simulink model "untitled"  (R2024b)
settings: Solver=VariableStepAuto  StartTime=0.0  StopTime=10.0  RelTol=1e-3
settings Model: Creator=yugan  LastModifiedBy=yugan
settings DebuggingCC: AlgebraicLoopMsg=none

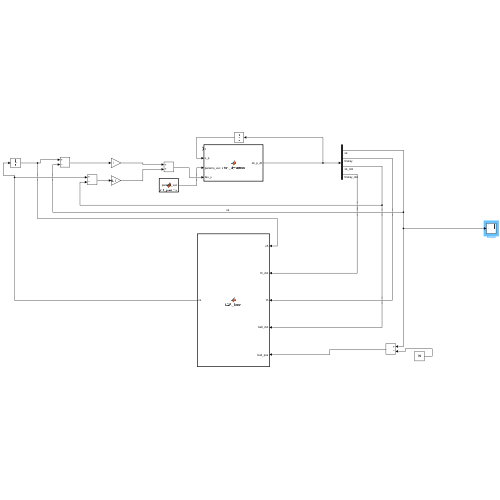
[thumbnail: Simulink's stored preview of the top-level diagram]
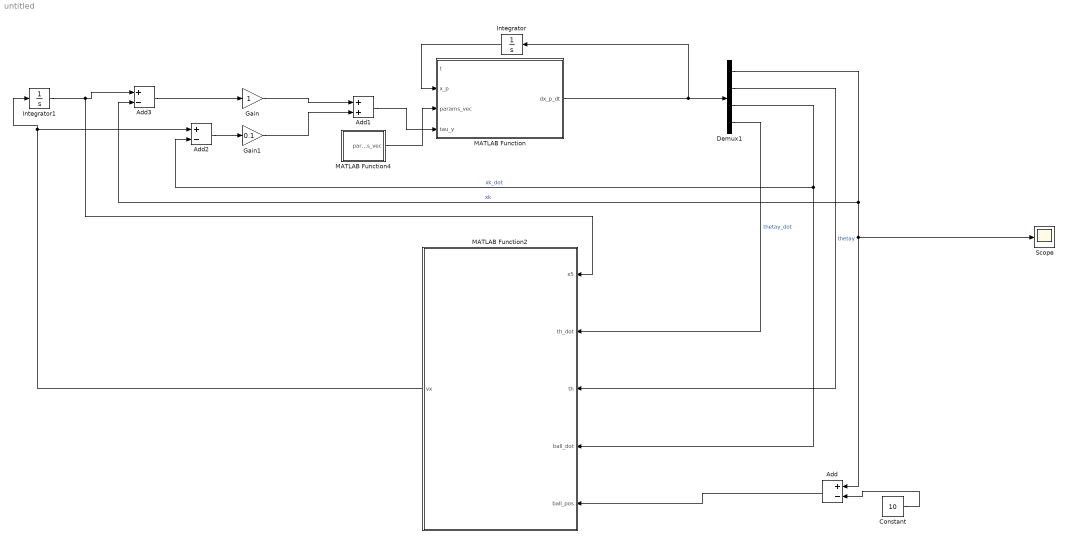
== system untitled ==
  Add : Sum  Inputs=+-
  Add1 : Sum
  Add2 : Sum  Inputs=+-
  Add3 : Sum  Inputs=+-
  Constant : Constant  Value=10
  Demux1 : Demux
  Gain : Gain
  Gain1 : Gain  Gain=0.1
  Integrator : Integrator  InitialCondition=[0; 0; 0; 0]
  Integrator1 : Integrator
  MATLAB Function : MATLAB Function  TreatAsAtomicUnit=on
  MATLAB Function2 : MATLAB Function  TreatAsAtomicUnit=on
  MATLAB Function4 : MATLAB Function  TreatAsAtomicUnit=on
  Scope : Scope
  wires:
  Integrator/1 -> MATLAB Function/2(x_p)
  MATLAB Function/1(dx_p_dt) -> Demux1/1, Integrator/1
  Demux1/1 -> Add3/2, Scope/1, Add/1  "xk"
  Add/1 -> MATLAB Function2/5(ball_pos)
  Constant/1 -> Add/2
  Demux1/2 -> MATLAB Function2/3(th)  "thetay"
  Demux1/3 -> MATLAB Function2/4(ball_dot), Add2/2  "xk_dot"
  Demux1/4 -> MATLAB Function2/2(th_dot)  "thetay_dot"
  Add1/1 -> MATLAB Function/4(tau_y)
  MATLAB Function4/1(params_vec) -> MATLAB Function/3(params_vec)
  Gain/1 -> Add1/1
  Gain1/1 -> Add1/2
  Add2/1 -> Gain1/1
  Add3/1 -> Gain/1
  MATLAB Function2/1(vx) -> Add2/1, Integrator1/1
  Integrator1/1 -> MATLAB Function2/1(x5), Add3/1

== matlab function untitled/MATLAB Function ==
  data: t input; dx_p_dt output; x_p input; params_vec input; tau_y input
function dx_p_dt = pitch_dynamics(t, x_p, params_vec, tau_y)
% pitch_dynamics.m
%
% 2-DOF dynamic model in the X–Z plane (pitch plane).
%
% State x_p = [x_k ; theta_y ; x_k_dot ; theta_y_dot]
% params_vec = 20×1 vector from init_params()
% Output dx_p_dt = state derivative (4×1)

%% ---------------------------------------------------------
% Unpack Parameters from Vector
%% ---------------------------------------------------------

mk  = params_vec(1);     % ball mass
Ik  = params_vec(2);     % ball inertia
ma  = params_vec(3);     % body mass
Ix  = params_vec(4);     % inertia about x
Iy  = params_vec(5);     % inertia about y
Iz  = params_vec(6);     % inertia about z
l   = params_vec(7);     % COM height
alpha_rad = params_vec(8); % zenith angle
rk  = params_vec(9);     % ball radius
rw  = params_vec(10);    % omniwheel radius
bx  = params_vec(11);
dx  = params_vec(12);
by  = params_vec(13);
dy  = params_vec(14);
bry = params_vec(15);
dry = params_vec(16);
brx = params_vec(17);
drx = params_vec(18);
g   = params_vec(19);    % gravity
k_motor = params_vec(20);

% Keep original notation
I_k_param = Ik;
I_w = Iy;    % consistent with roll dynamics formulation


%% ---------------------------------------------------------
% Extract State Variables
%% ---------------------------------------------------------

x_k         = x_p(1);
theta_y     = x_p(2);
x_k_dot     = x_p(3);
theta_y_dot = x_p(4);

q_y_dot = [x_k_dot ; theta_y_dot];


%% ---------------------------------------------------------
% Mass Matrix M(q)   (Eq. 8)
%% ---------------------------------------------------------

M11 = mk + (I_k_param / rk^2) + ma + ...
      (3*I_w*cos(alpha_rad)^2) / (2*rw^2);

M12 =   ma*l*cos(theta_y) ...
      - (3*I_w*cos(alpha_rad)^2)/(2*rw^2) * rk;

M21 = M12;

M22 = ma*l^2 + ...
      (3*I_w*rk^2*cos(alpha_rad)^2)/(2*rw^2) + Iy;

M_y = [M11 M12; M21 M22];


%% ---------------------------------------------------------
% Coriolis–Centrifugal Vector
%% ---------------------------------------------------------

C_y = [ 0                            -ma*l*theta_y_dot*sin(theta_y);
        0                             0 ];


%% ---------------------------------------------------------
% Gravity Vector
%% ---------------------------------------------------------

G_y = [0;
       -ma*g*l*sin(theta_y)];


%% ---------------------------------------------------------
% Friction Vector (ignored)
%% ---------------------------------------------------------

D_y = [0; 0];


%% ---------------------------------------------------------
% Input Torque Vector
%% ---------------------------------------------------------

Q_y = [ -(1/rw) * tau_y ;
         (rk/rw) * tau_y ];


%% ---------------------------------------------------------
% Solve q¨ = M⁻¹ (Q – C q̇ – D – G)
%% ---------------------------------------------------------

q_y_ddot = M_y \ (Q_y - C_y*q_y_dot - D_y - G_y);


%% ---------------------------------------------------------
% Output State Derivatives
%% ---------------------------------------------------------

dx_p_dt = [ x_k_dot ;
            theta_y_dot ;
            q_y_ddot(1) ;
            q_y_ddot(2) ];

end

== matlab function untitled/MATLAB Function4 ==
  data: params_vec output size=[20 1]
function params_vec = init_params()
% init_params.m
% Returns parameters as a 20×1 vector (NO STRUCT)

mk  = 19.6;                   % (1) ball mass
Ik  = 0.38;                   % (2) ball inertia
ma  = 68;                     % (3) body mass
Ix  = 12.1;                   % (4) body inertia x
Iy  = 11.67;                  % (5) body inertia y
Iz  = 1.08;                   % (6) body inertia z
l   = 0.38;                   % (7) COM height
a   = deg2rad(65.5);          % (8) zenith angle
rk  = 0.22;                   % (9) ball radius
rw  = 0.10;                   % (10) omniwheel radius
bx  = 0.10;                   % (11) viscous friction xz
dx  = 0.01;                   % (12) coulomb friction xz
by  = 0.10;                   % (13) viscous friction yz
dy  = 0.01;                   % (14) coulomb friction yz
bry = 0.12;                   % (15) body/ball viscous xz
dry = 0.02;                   % (16) coulomb xz
brx = 0.12;                   % (17) body/ball viscous yz
drx = 0.02;                   % (18) coulomb yz
g   = 9.81;                   % (19) gravity
k_motor = 1;                  % (20) motor constant


% Return as vector
params_vec = [
    mk; Ik; ma; Ix; Iy; Iz;
    l; a; rk; rw;
    bx; dx; by; dy;
    bry; dry; brx; drx;
    g; k_motor
];
end

== matlab function untitled/MATLAB Function2 ==
  data: x5 input; th_dot input; th input; ball_dot input; ball_pos input; vx output size=[1]
function vx  = LQR_Block(x5, th_dot, th, ball_dot, ball_pos)
%(x5, th, th_dot, )
% ========================================================================
%   REAL-TIME LQR CONTROLLER BLOCK
%   Applies pre-calculated gains Kr and Kp to the system states.
%
%   This block EXPECTS 'Kr' and 'Kp' to be passed in as parameters.
% ========================================================================

%% ------------------------------------------------------------
% BUILD STATE VECTORS
% **FIXED**: Swapped states back. Roll (y/2) and Pitch (x/1)
%            Please verify th(1) vs th(2) matches your setup.
%            Commonly: th(1)=pitch, th(2)=roll
%% ------------------------------------------------------------

  % example row
Kp = [-3.27, 4.01, 29.07, 8.54, 5.72];  % example row



xp = [ th;         % Pitch angle
       th_dot;     % Pitch rate
       ball_pos;   % Ball Y position (relative to pitch)
       ball_dot;   % Ball Y velocity
       x5          % Pitch integral term
       ];

%% ------------------------------------------------------------
% CONTROL LAWS (Simple multiplication)
%% ------------------------------------------------------------
 % Roll command
vx = -Kp * xp;   % Pitch command
end
